simulink model "Equation"  (Simulink 8.0)
settings: Solver=ode45  StartTime=0.0  StopTime=10.0  RelTol=1e-3
InitFcn:
  | a1=2;
  | a2=-3;
  | a3=-1;
  | a4=1;
  | a5=5;
  | a6=4;
  | a7=-6;
  | a8=1;
  | a9=2;
  | K1=-8;
  | K2=-7;
  | K3=5;
libraries: simulink x6
settings Model: Creator=Faradars  LastModifiedBy=Faradars

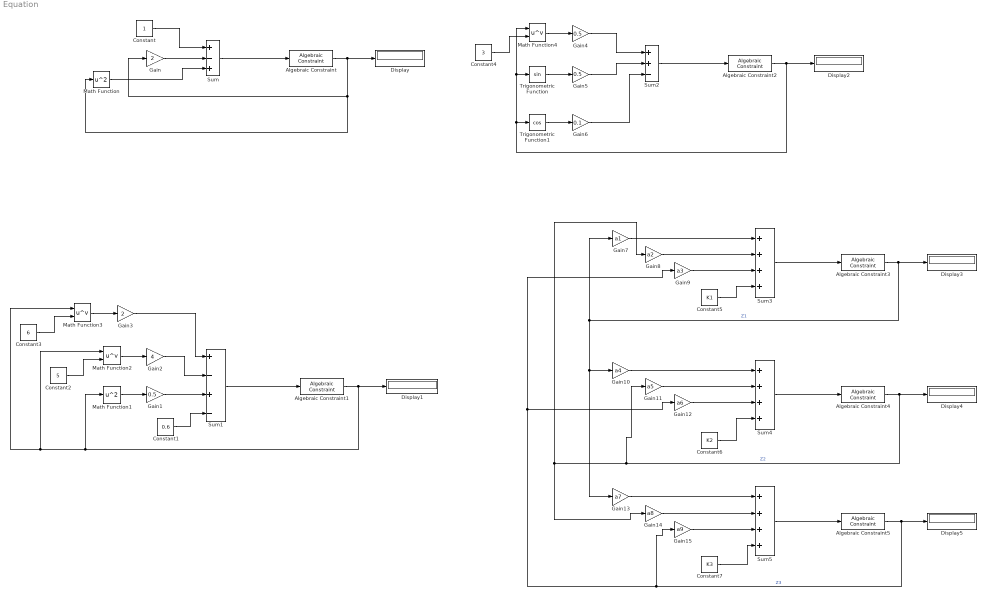
== system Equation ==
  Algebraic Constraint{,1..5} (6 alike) : simulink/Math Operations/Algebraic Constraint  z0=0
  Constant : Constant
  Constant1 : Constant  Value=0.6
  Constant2 : Constant  Value=5
  Constant3 : Constant  Value=6
  Constant4 : Constant  Value=3
  Constant5 : Constant  Value=K1
  Constant6 : Constant  Value=K2
  Constant7 : Constant  Value=K3
  Display{,1..5} (6 alike) : Display
  Gain : Gain  Gain=2
  Gain1 : Gain  Gain=0.5
  Gain10 : Gain  Gain=a4
  Gain11 : Gain  Gain=a5
  Gain12 : Gain  Gain=a6
  Gain13 : Gain  Gain=a7
  Gain14 : Gain  Gain=a8
  Gain15 : Gain  Gain=a9
  Gain2 : Gain  Gain=4
  Gain3 : Gain  Gain=2
  Gain4 : Gain  Gain=0.5
  Gain5 : Gain  Gain=0.5
  Gain6 : Gain  Gain=0.1
  Gain7 : Gain  Gain=a1
  Gain8 : Gain  Gain=a2
  Gain9 : Gain  Gain=a3
  Math Function : Math  Operator=square  SaturateOnIntegerOverflow=on
  Math Function1 : Math  Operator=square  SaturateOnIntegerOverflow=on
  Math Function2 : Math  Operator=pow  SaturateOnIntegerOverflow=on
  Math Function3 : Math  Operator=pow  SaturateOnIntegerOverflow=on
  Math Function4 : Math  Operator=pow  SaturateOnIntegerOverflow=on
  Sum : Sum  Inputs=+-+
  Sum1 : Sum  Inputs=+-+-
  Sum2 : Sum  Inputs=++-
  Sum3 : Sum  Inputs=++++
  Sum4 : Sum  Inputs=++++
  Sum5 : Sum  Inputs=++++
  Trigonometric Function : Trigonometry
  Trigonometric Function1 : Trigonometry  Operator=cos
  wires:
  Algebraic Constraint/1 -> Math Function/1, Gain/1, Display/1
  Sum/1 -> Algebraic Constraint/1
  Constant/1 -> Sum/1
  Gain/1 -> Sum/2
  Math Function/1 -> Sum/3
  Sum1/1 -> Algebraic Constraint1/1
  Constant1/1 -> Sum1/4
  Math Function1/1 -> Gain1/1
  Gain1/1 -> Sum1/3
  Math Function2/1 -> Gain2/1
  Constant2/1 -> Math Function2/2
  Gain2/1 -> Sum1/2
  Algebraic Constraint1/1 -> Math Function3/1, Math Function2/1, Math Function1/1, Display1/1
  Math Function3/1 -> Gain3/1
  Constant3/1 -> Math Function3/2
  Gain3/1 -> Sum1/1
  Algebraic Constraint2/1 -> Math Function4/1, Trigonometric Function/1, Trigonometric Function1/1, Display2/1
  Sum2/1 -> Algebraic Constraint2/1
  Math Function4/1 -> Gain4/1
  Constant4/1 -> Math Function4/2
  Gain4/1 -> Sum2/1
  Gain5/1 -> Sum2/2
  Trigonometric Function/1 -> Gain5/1
  Trigonometric Function1/1 -> Gain6/1
  Gain6/1 -> Sum2/3
  Algebraic Constraint3/1 -> Gain7/1, Gain13/1, Gain10/1, Display3/1  "Z1"
  Sum3/1 -> Algebraic Constraint3/1
  Algebraic Constraint4/1 -> Gain11/1, Gain8/1, Gain14/1, Display4/1  "Z2"
  Sum4/1 -> Algebraic Constraint4/1
  Algebraic Constraint5/1 -> Gain15/1, Gain9/1, Gain12/1, Display5/1  "Z3"
  Sum5/1 -> Algebraic Constraint5/1
  Constant5/1 -> Sum3/4
  Constant7/1 -> Sum5/4
  Constant6/1 -> Sum4/4
  Gain7/1 -> Sum3/1
  Gain8/1 -> Sum3/2
  Gain9/1 -> Sum3/3
  Gain10/1 -> Sum4/1
  Gain11/1 -> Sum4/2
  Gain12/1 -> Sum4/3
  Gain13/1 -> Sum5/1
  Gain14/1 -> Sum5/2
  Gain15/1 -> Sum5/3
